simulink model "CITRIS2"  (Simulink 7.4)
settings: Solver=FixedStepDiscrete  StartTime=0  StopTime=25  FixedStep=1  MaxStep=1  RelTol=1e-3
values from neighbouring files (symbols this model uses):
  mdot = [mdot controlInputHistory{i}(1,:)']    [CITRISBLOMSimulation.m]
  mdotmax = 740    [CITRISBLOMSimulation.m]
  mdotmin = 220    [CITRISBLOMSimulation.m]
  model =     [model.mat]
  T0 = 21    [CITRISBLOMSimulation.m]
  vlv = [vlv controlInputHistory{i}(2,:)']    [CITRISBLOMSimulation.m]
undefined symbols (not defined in the file or in its folder): i, mdotTk, mdotvlv, mdotvlvk, Tk, TmaxSlack, TmaxV, TminSlack, TminV, wk, wk_1, wk_2
libraries: BLOM_Lib x18
settings Model: Creator=vichik  LastModifiedBy=Kyle
settings OptimizationCC: InitFltsAndDblsToZero=on

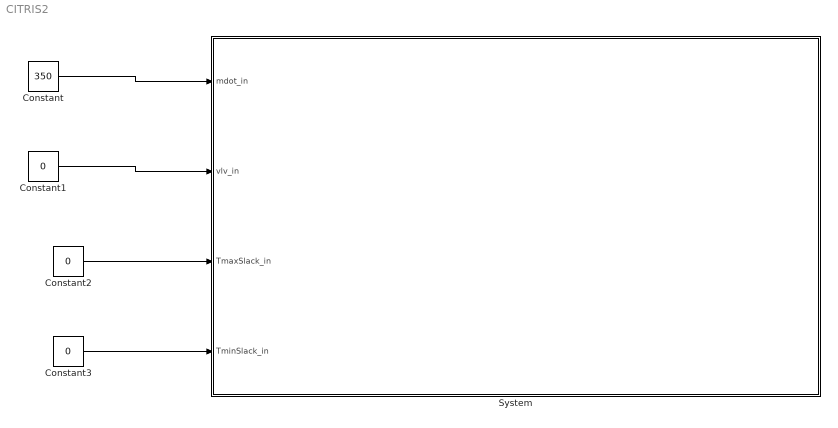
== system CITRIS2 ==
  Constant : Constant  Value=350
  Constant1 : Constant  Value=0
  Constant2 : Constant  Value=0
  Constant3 : Constant  Value=0
  System : Subsystem
  wires:
  Constant/1 -> System/1(mdot_in)
  Constant1/1 -> System/2(vlv_in)
  Constant2/1 -> System/3(TmaxSlack_in)
  Constant3/1 -> System/4(TminSlack_in)

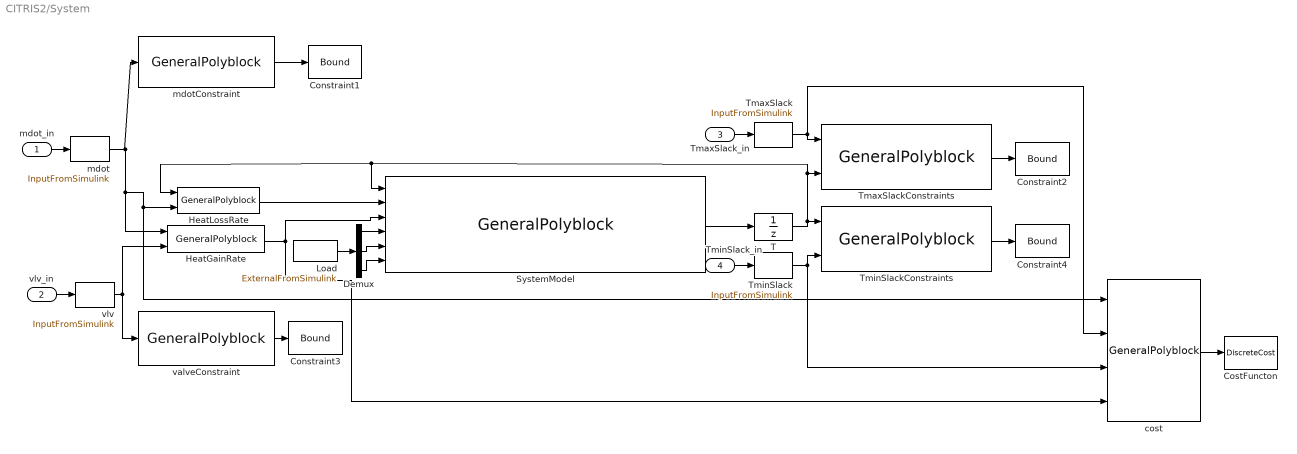
== system CITRIS2/System ==
  mdot_in : Inport
  vlv_in : Inport  Port=2
  TmaxSlack_in : Inport  Port=3
  TminSlack_in : Inport  Port=4
  Constraint{1..4} (4 alike) : BLOM_Lib/Bound  SystemSampleTime=-1  ub=0  lb=-inf  initial_step=on  intermediate_step=on  final_step=on
  CostFuncton : BLOM_Lib/DiscreteCost  SystemSampleTime=-1  initial_step=on  intermediate_step=on  final_step=on
  Demux : Demux  Outputs=3
  HeatGainRate : BLOM_Lib/GeneralPolyblock  SystemSampleTime=-1  P_f="[1  1  ]"  K_f=[1 ]  P_g=[0 0]  K_g=1  inputs=mdot,vlv  inputScalar=on  outputScalar=on
  HeatLossRate : BLOM_Lib/GeneralPolyblock  SystemSampleTime=-1  P_f="[1  1  ]"  K_f=[1 ]  P_g=[0 0]  K_g=1  inputs=Tk,mdot  inputScalar=on  outputScalar=on
  Load : BLOM_Lib/ExternalFromSimulink  SystemSampleTime=-1  interpType=Zero-Order Hold
  SystemModel : BLOM_Lib/GeneralPolyblock  SystemSampleTime=-1  P_f=[1 0 0 0 0 0;0 1 0 0 0 0;0 0 1 0 0 0;0 0 0 1 0 0;0 0 0 0 1 0;0 0 0 0 0 1;0 0 0 0 0 0]  K_f=[model{i}.A model{i}.B2 model{i}.B1 model{i}.W(1) model{i}.W(2) model{i}.W(3) model{i}.C]  P_g=[0 0 0 0 0 0]  K_g=1  inputs=Tk,mdotTk,mdotvlvk,wk,wk_1,wk_2  inputScalar=on  outputScalar=on
  T : UnitDelay  X0=T0  SampleTime=-1
  TmaxSlack : BLOM_Lib/InputFromSimulink  SystemSampleTime=-1  interpType=Zero-Order Hold
  TmaxSlackConstraints : BLOM_Lib/GeneralPolyblock  SystemSampleTime=-1  P_f=[0 1;1 0;0 0]  K_f=[1 -1 -22;0 -1 0]  P_g=[0 0]  K_g=1  inputs=TmaxSlack,Tk  inputScalar=on  outputScalar=off
  TminSlack : BLOM_Lib/InputFromSimulink  SystemSampleTime=-1  interpType=Zero-Order Hold
  TminSlackConstraints : BLOM_Lib/GeneralPolyblock  SystemSampleTime=-1  P_f=[1 0;0 1;0 0]  K_f=[-1 -1 20;0 -1 0]  P_g=[0 0]  K_g=1  inputs=Tk,TminSlack  inputScalar=on  outputScalar=off
  cost : BLOM_Lib/GeneralPolyblock  SystemSampleTime=-1  P_f=[0 0 1 0;0 1 0 0;2 0 0 0;0 0 0 1]  K_f=[1 1 1e-6 0.01*1e-5]  P_g=[0 0 0 0]  K_g=1  inputs=mdot,TmaxV,TminV,mdotvlv  inputScalar=on  outputScalar=on
  mdot : BLOM_Lib/InputFromSimulink  SystemSampleTime=-1  interpType=Zero-Order Hold
  mdotConstraint : BLOM_Lib/GeneralPolyblock  SystemSampleTime=-1  P_f="[1  ;  0 ]"  K_f=[1 -mdotmax; -1 mdotmin]  P_g="[0  ]"  K_g=1  inputs=mdot  inputScalar=on  outputScalar=off
  valveConstraint : BLOM_Lib/GeneralPolyblock  SystemSampleTime=-1  P_f=[1;0]  K_f="[1 -100; -1  0]"  P_g=[0]  K_g=1  inputs=vlv  inputScalar=on  outputScalar=off
  vlv : BLOM_Lib/InputFromSimulink  SystemSampleTime=-1  interpType=Zero-Order Hold
  wires:
  T/1 -> TmaxSlackConstraints/2, HeatLossRate/1, SystemModel/1, TminSlackConstraints/1
  mdot/1 -> HeatGainRate/1, HeatLossRate/2, cost/1, mdotConstraint/1
  cost/1 -> CostFuncton/1
  mdot_in/1 -> mdot/1
  mdotConstraint/1 -> Constraint1/1
  vlv_in/1 -> vlv/1
  vlv/1 -> HeatGainRate/2, valveConstraint/1
  valveConstraint/1 -> Constraint3/1
  HeatGainRate/1 -> SystemModel/3, cost/4
  TmaxSlackConstraints/1 -> Constraint2/1
  TminSlackConstraints/1 -> Constraint4/1
  TmaxSlack/1 -> TmaxSlackConstraints/1, cost/2
  SystemModel/1 -> T/1
  TminSlack/1 -> TminSlackConstraints/2, cost/3
  TmaxSlack_in/1 -> TmaxSlack/1
  TminSlack_in/1 -> TminSlack/1
  HeatLossRate/1 -> SystemModel/2
  Demux/1 -> SystemModel/4
  Demux/2 -> SystemModel/5
  Demux/3 -> SystemModel/6
  Load/1 -> Demux/1
